simulink subsystem "sonar"  (R2023b)
settings: Solver=VariableStepAuto  StartTime=0.0  StopTime=10.0  RelTol=1e-3
libraries: arduinolib x2
settings Model: Creator=Manuel  LastModifiedBy=Usuario_UMA

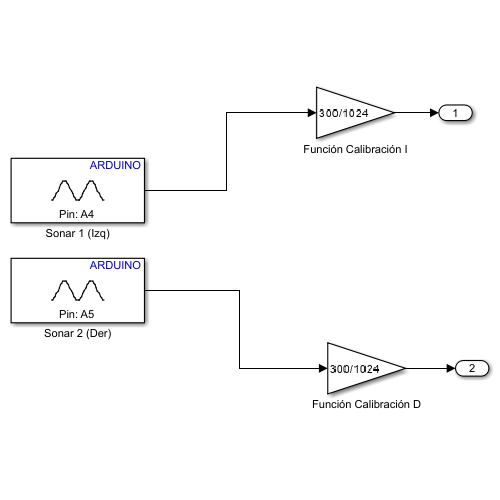
[thumbnail: Simulink's stored preview of the top-level diagram]
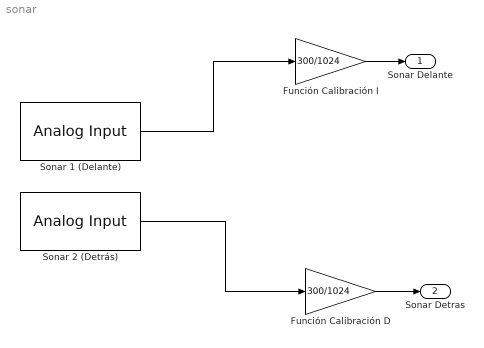
== system sonar ==
  Función Calibración D : Gain  Gain=300/1024
  Función Calibración I : Gain  Gain=300/1024
  Sonar 1 (Delante) : arduinolib/Analog Input  pinNumber=4  ReadResultsOnly=off  ConversionTriggerSource=Software  ExternalTriggerType=uint32( 0 )  OutputDataType=uint16  EnableConversionCompleteNotify=off  EnableOuputStatus=off  SampleTime=-1  blockPlatform=arduino
  Sonar 2 (Detrás) : arduinolib/Analog Input  pinNumber=5  ReadResultsOnly=off  ConversionTriggerSource=Software  ExternalTriggerType=uint32( 0 )  OutputDataType=uint16  EnableConversionCompleteNotify=off  EnableOuputStatus=off  SampleTime=-1  blockPlatform=arduino
  Sonar Delante : Outport
  Sonar Detras : Outport  Port=2
  wires:
  Sonar 2 (Detrás)/1 -> Función Calibración D/1
  Función Calibración D/1 -> Sonar Detras/1
  Función Calibración I/1 -> Sonar Delante/1
  Sonar 1 (Delante)/1 -> Función Calibración I/1
